simulink library "TriphaseHardwaremodule"  (R2019b)
settings: Solver=ode45  StartTime=0.0  StopTime=10.0  RelTol=1e-3
values from neighbouring files (symbols this model uses):
  ControlSampleTime = 1/8000    (= 0.000125)    [initTPHardware.m]
  HWSampleTime = ControlSampleTime / Oversample    [Sim_TP3_VSM_init.m]    (also in initTPHardware.m = 3.125e-05)
  L1 = 0    [initVirtualCircuit.m]
undefined symbols (not defined in the file or in its folder): C1, C2, C_cap, C_CM, C_damp, C_DC, DT, gcbh, Iac_bit, Iac_max, L2, L_CM, LCL, PWM_f, R_C1, R_C2, R_cap, R_damp, R_L1, R_L2, sps_rtmsupport, Vac_bit, Vac_max, Vdc_bit, Vdc_max
libraries: $bdroot x58, powerlib x46, triphase_hpc x7, powerlib_meascontrol x5, simulink x2
(part 2 of 3)

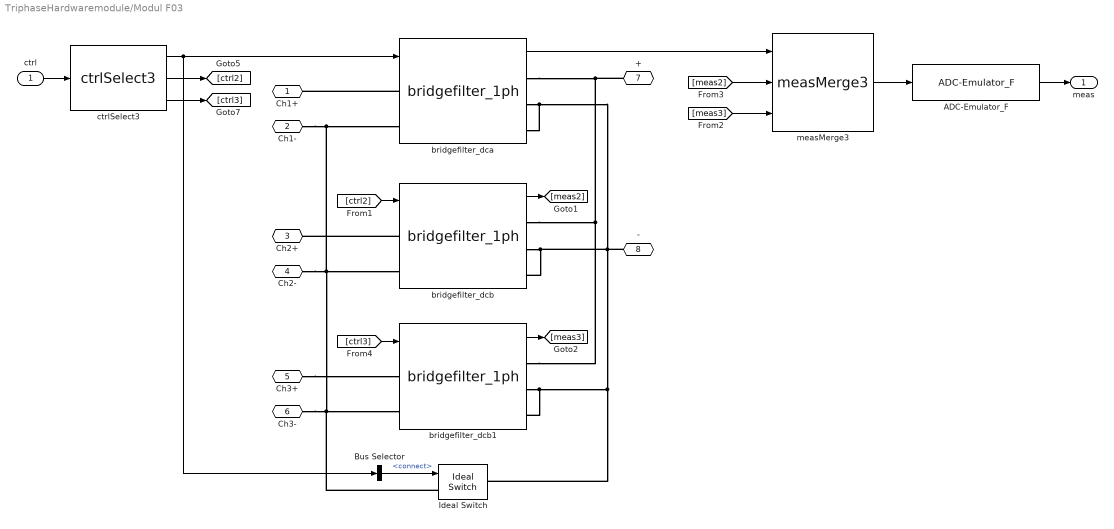
== system TriphaseHardwaremodule/Modul F03 ==
  ctrl : Inport
  ADC-Emulator_F : $bdroot/ADC-Emulator_F  ADC_Emulation=off  ControlSampleTime=ControlSampleTime  HWSampleTime=HWSampleTime  Vac_max=Vac_max  Vac_bit=Vac_bit  Iac_max=Iac_max  Iac_bit=Iac_bit  Vdc_max=Vdc_max  Vdc_bit=Vdc_bit
  Bus Selector : BusSelector  OutputSignals=connect
  Ideal Switch : powerlib/Power Electronics/Ideal Switch  Ron=0.001  Lon=0  IC=0  Rs=1e6  Cs=inf  Measurements=off
      settings: SourceProductName=Simscape Electrical
  bridgefilter_dca : $bdroot/bridgefilter_1ph  LCFilterChoice=LC  L1=L1  R_L1=R_L1  C1=C1  R_C1=R_C1  L2=L2  R_L2=R_L2  C2=C2  R_C2=R_C2  PWM_f=PWM_f  DT=DT
  bridgefilter_dcb : $bdroot/bridgefilter_1ph  LCFilterChoice=LC  L1=L1  R_L1=R_L1  C1=C1  R_C1=R_C1  L2=L2  R_L2=R_L2  C2=C2  R_C2=R_C2  PWM_f=PWM_f  DT=DT
  bridgefilter_dcb1 : $bdroot/bridgefilter_1ph  LCFilterChoice=LC  L1=L1  R_L1=R_L1  C1=C1  R_C1=R_C1  L2=L2  R_L2=R_L2  C2=C2  R_C2=R_C2  PWM_f=PWM_f  DT=DT
  ctrlSelect3 : $bdroot/ctrlSelect3
  measMerge3 : $bdroot/measMerge3
  Ch1+ : PMIOPort  Tag=PMCPort  Side=Left
  Ch1- : PMIOPort  Tag=PMCPort  Port=2  Side=Left
  Ch2+ : PMIOPort  Tag=PMCPort  Port=3  Side=Left
  Ch2- : PMIOPort  Tag=PMCPort  Port=4  Side=Left
  Ch3+ : PMIOPort  Tag=PMCPort  Port=5  Side=Left
  Ch3- : PMIOPort  Tag=PMCPort  Port=6  Side=Left
  + : PMIOPort  Tag=PMCPort  Port=7  Side=Right
  - : PMIOPort  Tag=PMCPort  Port=8  Side=Right
  meas : Outport  VectorParamsAs1DForOutWhenUnconnected=off
  wires:
  ADC-Emulator_F/1 -> meas/1
  measMerge3/1 -> ADC-Emulator_F/1
  Bus Selector/1 -> Ideal Switch/1  "<connect>"
  ctrlSelect3/1 -> bridgefilter_dca/1, Bus Selector/1
  bridgefilter_dcb/1 -> [meas2]
  bridgefilter_dca/1 -> measMerge3/1
  [meas2] -> measMerge3/2
  ctrl/1 -> ctrlSelect3/1
  ctrlSelect3/2 -> [ctrl2]
  [ctrl2] -> bridgefilter_dcb/1
  bridgefilter_dcb1/1 -> [meas3]
  [meas3] -> measMerge3/3
  ctrlSelect3/3 -> [ctrl3]
  [ctrl3] -> bridgefilter_dcb1/1
  connections:
  bridgefilter_dcb1/RConn2 -- bridgefilter_dcb1/RConn3 -- Ideal Switch/RConn1 -- -/RConn1 -- bridgefilter_dca/RConn3 -- bridgefilter_dca/RConn2 -- bridgefilter_dcb/RConn3 -- bridgefilter_dcb/RConn2
  +/RConn1 -- bridgefilter_dcb1/RConn1 -- bridgefilter_dcb/RConn1 -- bridgefilter_dca/RConn1
  bridgefilter_dcb/LConn1 -- Ch2+/RConn1
  bridgefilter_dca/LConn1 -- Ch1+/RConn1
  Ch3+/RConn1 -- bridgefilter_dcb1/LConn1
  Ch2-/RConn1 -- Ideal Switch/LConn1 -- Ch3-/RConn1 -- bridgefilter_dcb1/LConn2 -- bridgefilter_dcb/LConn2 -- Ch1-/RConn1 -- bridgefilter_dca/LConn2

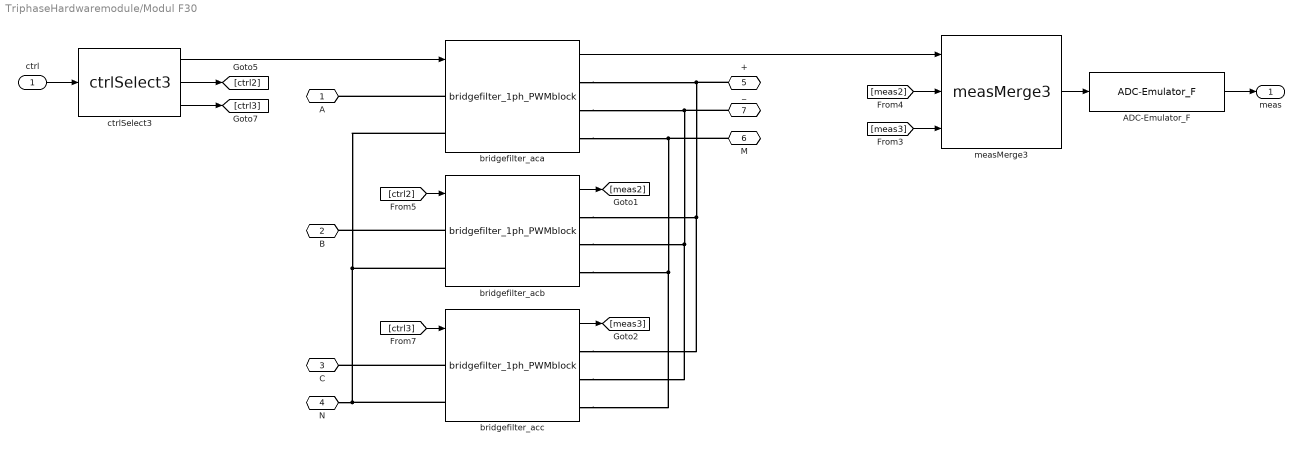
== system TriphaseHardwaremodule/Modul F30 ==
  ctrl : Inport
  ADC-Emulator_F : $bdroot/ADC-Emulator_F  ADC_Emulation=off  ControlSampleTime=ControlSampleTime  HWSampleTime=HWSampleTime  Vac_max=Vac_max  Vac_bit=Vac_bit  Iac_max=Iac_max  Iac_bit=Iac_bit  Vdc_max=Vdc_max  Vdc_bit=Vdc_bit
  bridgefilter_aca : $bdroot/bridgefilter_1ph_PWMblock  LCFilterChoice=LCLC  L1=L1  R_L1=R_L1  C1=C1  R_C1=R_C1  L2=L2  R_L2=R_L2  C2=C2  R_C2=R_C2  PWM_f=PWM_f  DT=DT  I_MAX=250  I_BACK=180
  bridgefilter_acb : $bdroot/bridgefilter_1ph_PWMblock  LCFilterChoice=LCLC  L1=L1  R_L1=R_L1  C1=C1  R_C1=R_C1  L2=L2  R_L2=R_L2  C2=C2  R_C2=R_C2  PWM_f=PWM_f  DT=DT  I_MAX=250  I_BACK=180
  bridgefilter_acc : $bdroot/bridgefilter_1ph_PWMblock  LCFilterChoice=LCLC  L1=L1  R_L1=R_L1  C1=C1  R_C1=R_C1  L2=L2  R_L2=R_L2  C2=C2  R_C2=R_C2  PWM_f=PWM_f  DT=DT  I_MAX=250  I_BACK=180
  ctrlSelect3 : $bdroot/ctrlSelect3  SystemSampleTime=-1
  measMerge3 : $bdroot/measMerge3  SystemSampleTime=-1
  A : PMIOPort  Tag=PMCPort  Side=Left
  B : PMIOPort  Tag=PMCPort  Port=2  Side=Left
  C : PMIOPort  Tag=PMCPort  Port=3  Side=Left
  N : PMIOPort  Tag=PMCPort  Port=4  Side=Left
  + : PMIOPort  Tag=PMCPort  Port=5  Side=Right
  M : PMIOPort  Tag=PMCPort  Port=6  Side=Right
  _ : PMIOPort  Tag=PMCPort  Port=7  Side=Right
  meas : Outport  VectorParamsAs1DForOutWhenUnconnected=off
  wires:
  measMerge3/1 -> ADC-Emulator_F/1
  ADC-Emulator_F/1 -> meas/1
  ctrlSelect3/1 -> bridgefilter_aca/1
  [ctrl3] -> bridgefilter_acc/1
  [ctrl2] -> bridgefilter_acb/1
  ctrlSelect3/2 -> [ctrl2]
  ctrlSelect3/3 -> [ctrl3]
  ctrl/1 -> ctrlSelect3/1
  [meas2] -> measMerge3/2
  bridgefilter_acc/1 -> [meas3]
  bridgefilter_acb/1 -> [meas2]
  [meas3] -> measMerge3/3
  bridgefilter_aca/1 -> measMerge3/1
  connections:
  bridgefilter_acc/LConn2 -- N/RConn1 -- bridgefilter_acb/LConn2 -- bridgefilter_aca/LConn2
  _/RConn1 -- bridgefilter_aca/RConn2 -- bridgefilter_acc/RConn2 -- bridgefilter_acb/RConn2
  bridgefilter_aca/RConn3 -- M/RConn1 -- bridgefilter_acc/RConn3 -- bridgefilter_acb/RConn3
  bridgefilter_aca/RConn1 -- +/RConn1 -- bridgefilter_acc/RConn1 -- bridgefilter_acb/RConn1
  bridgefilter_acc/LConn1 -- C/RConn1
  bridgefilter_acb/LConn1 -- B/RConn1
  bridgefilter_aca/LConn1 -- A/RConn1

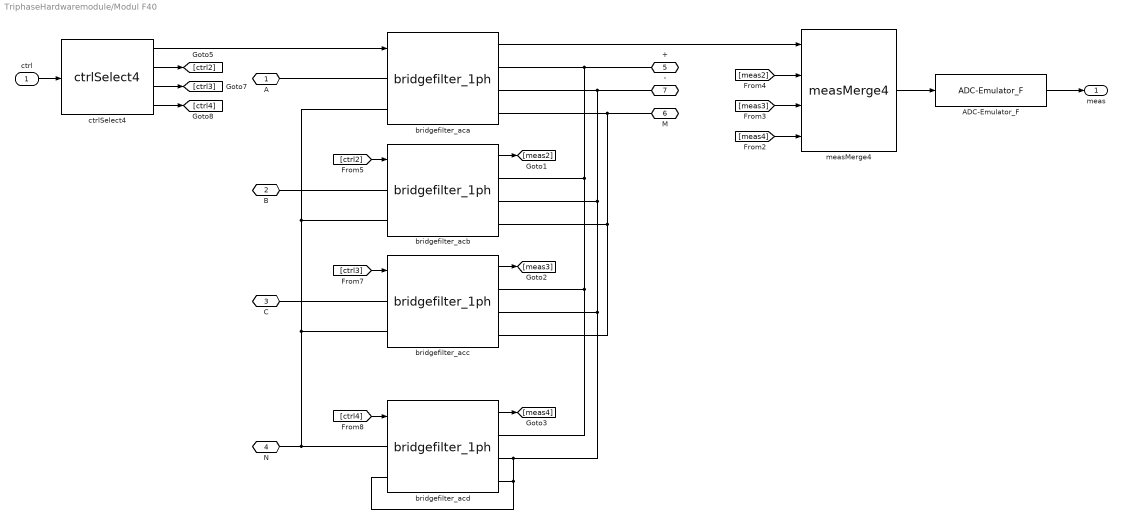
== system TriphaseHardwaremodule/Modul F40 ==
  ctrl : Inport
  ADC-Emulator_F : $bdroot/ADC-Emulator_F  ADC_Emulation=off  ControlSampleTime=ControlSampleTime  HWSampleTime=HWSampleTime  Vac_max=Vac_max  Vac_bit=Vac_bit  Iac_max=Iac_max  Iac_bit=Iac_bit  Vdc_max=Vdc_max  Vdc_bit=Vdc_bit
  bridgefilter_aca : $bdroot/bridgefilter_1ph  LCFilterChoice=LC  L1=L1  R_L1=R_L1  C1=C1  R_C1=R_C1  L2=L2  R_L2=R_L2  C2=C2  R_C2=R_C2  PWM_f=PWM_f  DT=DT
  bridgefilter_acb : $bdroot/bridgefilter_1ph  LCFilterChoice=LC  L1=L1  R_L1=R_L1  C1=C1  R_C1=R_C1  L2=L2  R_L2=R_L2  C2=C2  R_C2=R_C2  PWM_f=PWM_f  DT=DT
  bridgefilter_acc : $bdroot/bridgefilter_1ph  LCFilterChoice=LC  L1=L1  R_L1=R_L1  C1=C1  R_C1=R_C1  L2=L2  R_L2=R_L2  C2=C2  R_C2=R_C2  PWM_f=PWM_f  DT=DT
  bridgefilter_acd : $bdroot/bridgefilter_1ph  LCFilterChoice=LC  L1=L1  R_L1=R_L1  C1=C1  R_C1=R_C1  L2=L2  R_L2=R_L2  C2=C2  R_C2=R_C2  PWM_f=PWM_f  DT=DT
  ctrlSelect4 : $bdroot/ctrlSelect4
  measMerge4 : $bdroot/measMerge4
  A : PMIOPort  Tag=PMCPort  Side=Left
  B : PMIOPort  Tag=PMCPort  Port=2  Side=Left
  C : PMIOPort  Tag=PMCPort  Port=3  Side=Left
  N : PMIOPort  Tag=PMCPort  Port=4  Side=Left
  + : PMIOPort  Tag=PMCPort  Port=5  Side=Right
  M : PMIOPort  Tag=PMCPort  Port=6  Side=Right
  - : PMIOPort  Tag=PMCPort  Port=7  Side=Right
  meas : Outport  VectorParamsAs1DForOutWhenUnconnected=off
  wires:
  ctrlSelect4/1 -> bridgefilter_aca/1
  [ctrl4] -> bridgefilter_acd/1
  [ctrl3] -> bridgefilter_acc/1
  [ctrl2] -> bridgefilter_acb/1
  ctrlSelect4/2 -> [ctrl2]
  ctrlSelect4/3 -> [ctrl3]
  ctrlSelect4/4 -> [ctrl4]
  ctrl/1 -> ctrlSelect4/1
  measMerge4/1 -> ADC-Emulator_F/1
  [meas2] -> measMerge4/2
  bridgefilter_acd/1 -> [meas4]
  bridgefilter_acc/1 -> [meas3]
  bridgefilter_acb/1 -> [meas2]
  [meas4] -> measMerge4/4
  [meas3] -> measMerge4/3
  bridgefilter_aca/1 -> measMerge4/1
  ADC-Emulator_F/1 -> meas/1
  connections:
  bridgefilter_acc/LConn2 -- N/RConn1 -- bridgefilter_acd/LConn1 -- bridgefilter_acb/LConn2 -- bridgefilter_aca/LConn2
  bridgefilter_acc/LConn1 -- C/RConn1
  bridgefilter_acb/LConn1 -- B/RConn1
  bridgefilter_aca/LConn1 -- A/RConn1
  bridgefilter_aca/RConn1 -- bridgefilter_acd/RConn1 -- bridgefilter_acc/RConn1 -- bridgefilter_acb/RConn1 -- +/RConn1
  -/RConn1 -- bridgefilter_aca/RConn2 -- bridgefilter_acb/RConn2 -- bridgefilter_acd/LConn2 -- bridgefilter_acd/RConn3 -- bridgefilter_acd/RConn2 -- bridgefilter_acc/RConn2
  M/RConn1 -- bridgefilter_acc/RConn3 -- bridgefilter_acb/RConn3 -- bridgefilter_aca/RConn3

== system TriphaseHardwaremodule/Modul M30 ==
  ctrl : Inport
  ADC-Emulator_M : $bdroot/ADC-Emulator_M  ADC_Emulation=off  ControlSampleTime=ControlSampleTime  HWSampleTime=HWSampleTime  Vac_max=Vac_max  Vac_bit=Vac_bit  Iac_max=Iac_max  Iac_bit=Iac_bit  Vdc_max=Vdc_max  Vdc_bit=Vdc_bit
  B6 Brücke : Subsystem  InitFcn=|  Variant=on
      | if ~exist('SimulationMode','var')
      | SimulationMode = 1;
      | end
      settings: AttributesFormatString=%<ActiveVariant>
  Bus Creator : BusCreator  Inputs=2
  Bus Selector : BusSelector  OutputSignals=pwm
  Decoupling Resistance : powerlib/Elements/Three-Phase Parallel RLC Branch  LConnTagsString=A|B|C  RConnTagsString=A|B|C  BranchType=R  Resistance=0.0001  Inductance=1e-3  Capacitance=1e-6  Measurements=None
      settings: SourceProductName=Simscape Electrical  SourceProductBaseCode=PS
  Three-Phase I-Measurement (right to left = positive) : powerlib/Measurements/Three-Phase V-I Measurement  VoltageMeasurement=no  SetLabelV=off  LabelV=Vabc  Vpu=off  VpuLL=off  CurrentMeasurement=yes  SetLabelI=off  LabelI=I_out  Ipu=off  Pbase=100e6  Vbase=500e3  OutputType=Complex  PhasorSimulation=off  PSBequivalent=0
      settings: SourceProductName=Simscape Electrical
  Voltage Measurement : powerlib/Measurements/Voltage Measurement  PhasorSimulation=off  OutputType=Complex  PSBequivalent=0
      settings: SourceProductName=Simscape Electrical
  + : PMIOPort  Side=Right
  - : PMIOPort  Port=2  Side=Right
  A : PMIOPort  Port=3  Side=Left
  B : PMIOPort  Port=4  Side=Left
  C : PMIOPort  Port=5  Side=Left
  meas : Outport  VectorParamsAs1DForOutWhenUnconnected=off
  wires:
  Three-Phase I-Measurement (right to left = positive)/1 -> Bus Creator/1  "meas_i_inverter"
  Voltage Measurement/1 -> Bus Creator/2  "meas_u_dc"
  ctrl/1 -> Bus Selector/1
  Bus Selector/1 -> B6 Brücke/1(DutyCycle)  "<pwm>"
  Bus Creator/1 -> ADC-Emulator_M/1
  ADC-Emulator_M/1 -> meas/1
  connections:
  -/RConn1 -- Voltage Measurement/LConn2 -- B6 Brücke/RConn2
  B6 Brücke/RConn1 -- Voltage Measurement/LConn1 -- +/RConn1
  Three-Phase I-Measurement (right to left = positive)/LConn1 -- B6 Brücke/LConn1
  Three-Phase I-Measurement (right to left = positive)/LConn2 -- B6 Brücke/LConn2
  Three-Phase I-Measurement (right to left = positive)/LConn3 -- B6 Brücke/LConn3
  Decoupling Resistance/RConn3 -- Three-Phase I-Measurement (right to left = positive)/RConn3
  Decoupling Resistance/RConn2 -- Three-Phase I-Measurement (right to left = positive)/RConn2
  Decoupling Resistance/RConn1 -- Three-Phase I-Measurement (right to left = positive)/RConn1
  A/RConn1 -- Decoupling Resistance/LConn1
  B/RConn1 -- Decoupling Resistance/LConn2
  C/RConn1 -- Decoupling Resistance/LConn3

== system TriphaseHardwaremodule/PMXXF03C ==
  Setpoints : Inport
  Bus Creator : BusCreator  Inputs=1
  Bus Selector : BusSelector  OutputSignals=preload,Inv1
  DC-Bus : $bdroot/DC-Bus  C_cap=C_cap  R_cap=R_cap
  Modul F03 : $bdroot/Modul F03  Leistungsklasse=Custom  LCFilterChoice=LC  L1=L1  R_L1=R_L1  C1=C1  R_C1=R_C1  L2=L2  R_L2=R_L2  C2=C2  R_C2=R_C2  PWM_f=PWM_f  DT=DT  ADC_Emulation=off  ControlSampleTime=ControlSampleTime  HWSampleTime=HWSampleTime  Vac_max=Vac_max  Vac_bit=Vac_bit  Iac_max=Iac_max  Iac_bit=Iac_bit  Vdc_max=Vdc_max  Vdc_bit=Vdc_bit
  A1+ : PMIOPort  Tag=PMCPort  Side=Left
  A1- : PMIOPort  Tag=PMCPort  Port=2  Side=Left
  B1+ : PMIOPort  Tag=PMCPort  Port=3  Side=Left
  B1- : PMIOPort  Tag=PMCPort  Port=4  Side=Left
  C1+ : PMIOPort  Tag=PMCPort  Port=5  Side=Left
  C1- : PMIOPort  Tag=PMCPort  Port=6  Side=Left
  A_rect : PMIOPort  Tag=PMCPort  Port=7  Side=Right
  B_rect : PMIOPort  Tag=PMCPort  Port=8  Side=Right
  C_rect : PMIOPort  Tag=PMCPort  Port=9  Side=Right
  ZWK+ : PMIOPort  Tag=PMCPort  Port=10  Side=Right
  ZWK- : PMIOPort  Tag=PMCPort  Port=11  Side=Right
  Measurements : Outport  VectorParamsAs1DForOutWhenUnconnected=off
  wires:
  Setpoints/1 -> Bus Selector/1
  Bus Selector/1 -> DC-Bus/1  "<preload>"
  Bus Creator/1 -> Measurements/1
  Modul F03/1 -> Bus Creator/1  "Inv1"
  Bus Selector/2 -> Modul F03/1  "<Inv1>"
  connections:
  Modul F03/RConn1 -- DC-Bus/LConn4
  Modul F03/LConn1 -- A1+/RConn1
  DC-Bus/RConn1 -- A_rect/RConn1
  DC-Bus/RConn2 -- B_rect/RConn1
  DC-Bus/RConn3 -- C_rect/RConn1
  ZWK+/RConn1 -- DC-Bus/RConn4
  DC-Bus/RConn5 -- ZWK-/RConn1
  Modul F03/RConn2 -- DC-Bus/LConn6
  A1-/RConn1 -- Modul F03/LConn2
  B1+/RConn1 -- Modul F03/LConn3
  B1-/RConn1 -- Modul F03/LConn4
  C1+/RConn1 -- Modul F03/LConn5
  C1-/RConn1 -- Modul F03/LConn6

== system TriphaseHardwaremodule/PMXXF30C ==
  Setpoints : Inport
  Bus Creator : BusCreator  Inputs=1
  Bus Selector : BusSelector  OutputSignals=preload,Inv1
  DC-Bus : $bdroot/DC-Bus  C_cap=C_cap  R_cap=R_cap
  Modul F30 : $bdroot/Modul F30  Leistungsklasse=Custom  LCFilterChoice=LC  L1=L1  R_L1=R_L1  C1=C1  R_C1=R_C1  L2=L2  R_L2=R_L2  C2=C2  R_C2=R_C2  PWM_f=PWM_f  DT=DT  ADC_Emulation=off  ControlSampleTime=ControlSampleTime  HWSampleTime=HWSampleTime  Vac_max=Vac_max  Vac_bit=Vac_bit  Iac_max=Iac_max  Iac_bit=Iac_bit  Vdc_max=Vdc_max  Vdc_bit=Vdc_bit
  A1 : PMIOPort  Tag=PMCPort  Side=Left
  B1 : PMIOPort  Tag=PMCPort  Port=2  Side=Left
  C1 : PMIOPort  Tag=PMCPort  Port=3  Side=Left
  N1 : PMIOPort  Tag=PMCPort  Port=4  Side=Left
  A_rect : PMIOPort  Tag=PMCPort  Port=5  Side=Right
  B_rect : PMIOPort  Tag=PMCPort  Port=6  Side=Right
  C_rect : PMIOPort  Tag=PMCPort  Port=7  Side=Right
  ZWK+ : PMIOPort  Tag=PMCPort  Port=8  Side=Right
  ZWK- : PMIOPort  Tag=PMCPort  Port=9  Side=Right
  Measurements : Outport  VectorParamsAs1DForOutWhenUnconnected=off
  wires:
  Bus Selector/2 -> Modul F30/1  "<Inv1>"
  Setpoints/1 -> Bus Selector/1
  Bus Selector/1 -> DC-Bus/1  "<preload>"
  Bus Creator/1 -> Measurements/1
  Modul F30/1 -> Bus Creator/1  "Inv1"
  connections:
  Modul F30/LConn3 -- C1/RConn1
  Modul F30/LConn2 -- B1/RConn1
  Modul F30/LConn1 -- A1/RConn1
  DC-Bus/LConn1 -- Modul F30/RConn1
  DC-Bus/LConn2 -- Modul F30/RConn2
  DC-Bus/LConn3 -- Modul F30/RConn3
  DC-Bus/RConn3 -- C_rect/RConn1
  DC-Bus/RConn2 -- B_rect/RConn1
  DC-Bus/RConn1 -- A_rect/RConn1
  DC-Bus/RConn4 -- ZWK+/RConn1
  DC-Bus/RConn5 -- ZWK-/RConn1
  N1/RConn1 -- Modul F30/LConn4

== system TriphaseHardwaremodule/PMXXF30Cver270612 ==
  Setpoints : Inport
  Bus Creator : BusCreator  Inputs=2
  Bus Selector : BusSelector  OutputSignals=preload,Inv1
  DC-Bus : $bdroot/DC-Bus  C_cap=C_cap  R_cap=R_cap
  Modul F30 : $bdroot/Modul F30  Leistungsklasse=Custom  LCFilterChoice=LC  L1=L1  R_L1=R_L1  C1=C1  R_C1=R_C1  L2=L2  R_L2=R_L2  C2=C2  R_C2=R_C2  PWM_f=PWM_f  DT=DT  ADC_Emulation=off  ControlSampleTime=ControlSampleTime  HWSampleTime=HWSampleTime  Vac_max=Vac_max  Vac_bit=Vac_bit  Iac_max=Iac_max  Iac_bit=Iac_bit  Vdc_max=Vdc_max  Vdc_bit=Vdc_bit
  emptyMeasure : $bdroot/emptyMeasure
  A1 : PMIOPort  Tag=PMCPort  Side=Left
  B1 : PMIOPort  Tag=PMCPort  Port=2  Side=Left
  C1 : PMIOPort  Tag=PMCPort  Port=3  Side=Left
  N1 : PMIOPort  Tag=PMCPort  Port=4  Side=Left
  ZWK+ : PMIOPort  Tag=PMCPort  Port=5  Side=Right
  ZWK- : PMIOPort  Tag=PMCPort  Port=6  Side=Right
  Measurements : Outport  VectorParamsAs1DForOutWhenUnconnected=off
  wires:
  Bus Selector/1 -> DC-Bus/1  "<preload>"
  Setpoints/1 -> Bus Selector/1
  Bus Creator/1 -> Measurements/1
  Modul F30/1 -> Bus Creator/1  "Inv1"
  emptyMeasure/1 -> Bus Creator/2  "Inv2"
  Bus Selector/2 -> Modul F30/1  "<Inv1>"
  connections:
  DC-Bus/RConn1 -- Modul F30/LConn1 -- A1/RConn1
  DC-Bus/RConn2 -- B1/RConn1 -- Modul F30/LConn2
  DC-Bus/RConn3 -- Modul F30/LConn3 -- C1/RConn1
  ZWK-/RConn1 -- DC-Bus/RConn5
  ZWK+/RConn1 -- DC-Bus/RConn4
  Modul F30/RConn1 -- DC-Bus/LConn1
  Modul F30/RConn2 -- DC-Bus/LConn2
  Modul F30/RConn3 -- DC-Bus/LConn3
  N1/RConn1 -- Modul F30/LConn4

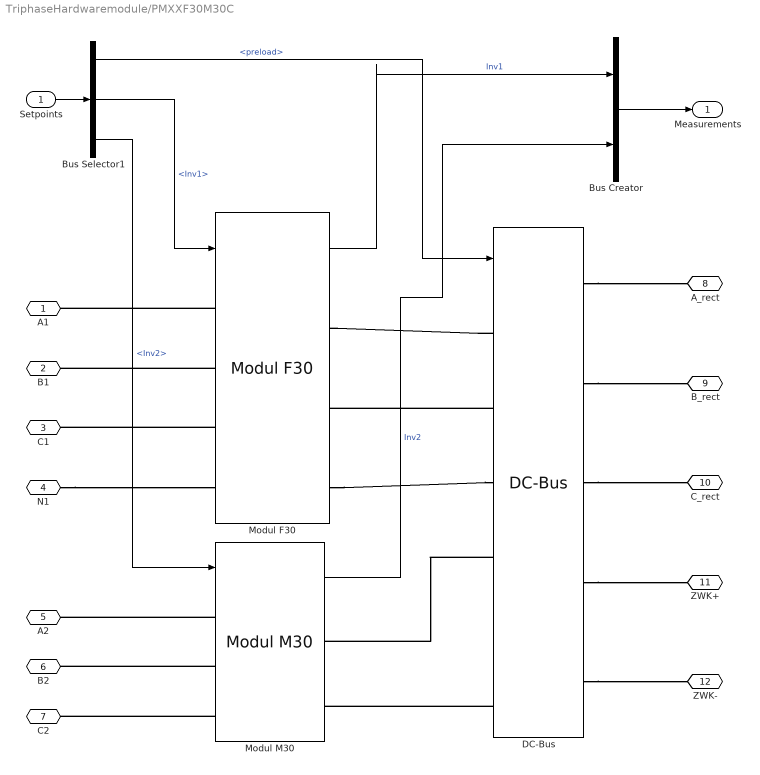
== system TriphaseHardwaremodule/PMXXF30M30C ==
  Setpoints : Inport
  Bus Creator : BusCreator  Inputs=2
  Bus Selector1 : BusSelector  OutputSignals=preload,Inv1,Inv2
  DC-Bus : $bdroot/DC-Bus  C_cap=C_cap  R_cap=R_cap
  Modul F30 : $bdroot/Modul F30  Leistungsklasse=Custom  LCFilterChoice=LC  L1=L1  R_L1=R_L1  C1=C1  R_C1=R_C1  L2=L2  R_L2=R_L2  C2=C2  R_C2=R_C2  PWM_f=PWM_f  DT=DT  ADC_Emulation=off  ControlSampleTime=ControlSampleTime  HWSampleTime=HWSampleTime  Vac_max=Vac_max  Vac_bit=Vac_bit  Iac_max=Iac_max  Iac_bit=Iac_bit  Vdc_max=Vdc_max  Vdc_bit=Vdc_bit
  Modul M30 : $bdroot/Modul M30  PWM_f=PWM_f  DT=DT
  A1 : PMIOPort  Tag=PMCPort  Side=Left
  B1 : PMIOPort  Tag=PMCPort  Port=2  Side=Left
  C1 : PMIOPort  Tag=PMCPort  Port=3  Side=Left
  N1 : PMIOPort  Tag=PMCPort  Port=4  Side=Left
  A2 : PMIOPort  Tag=PMCPort  Port=5  Side=Left
  B2 : PMIOPort  Tag=PMCPort  Port=6  Side=Left
  C2 : PMIOPort  Tag=PMCPort  Port=7  Side=Left
  A_rect : PMIOPort  Tag=PMCPort  Port=8  Side=Right
  B_rect : PMIOPort  Tag=PMCPort  Port=9  Side=Right
  C_rect : PMIOPort  Tag=PMCPort  Port=10  Side=Right
  ZWK+ : PMIOPort  Tag=PMCPort  Port=11  Side=Right
  ZWK- : PMIOPort  Tag=PMCPort  Port=12  Side=Right
  Measurements : Outport  VectorParamsAs1DForOutWhenUnconnected=off
  wires:
  Bus Selector1/3 -> Modul M30/1  "<Inv2>"
  Bus Selector1/2 -> Modul F30/1  "<Inv1>"
  Setpoints/1 -> Bus Selector1/1
  Modul F30/1 -> Bus Creator/1  "Inv1"
  Bus Selector1/1 -> DC-Bus/1  "<preload>"
  Bus Creator/1 -> Measurements/1
  Modul M30/1 -> Bus Creator/2  "Inv2"
  connections:
  Modul F30/LConn3 -- C1/RConn1
  Modul F30/LConn2 -- B1/RConn1
  Modul F30/LConn1 -- A1/RConn1
  Modul M30/LConn2 -- B2/RConn1
  Modul M30/LConn1 -- A2/RConn1
  Modul M30/LConn3 -- C2/RConn1
  DC-Bus/RConn3 -- C_rect/RConn1
  DC-Bus/RConn2 -- B_rect/RConn1
  DC-Bus/RConn1 -- A_rect/RConn1
  DC-Bus/RConn4 -- ZWK+/RConn1
  DC-Bus/RConn5 -- ZWK-/RConn1
  DC-Bus/LConn2 -- Modul F30/RConn2
  DC-Bus/LConn1 -- Modul F30/RConn1
  DC-Bus/LConn4 -- Modul M30/RConn1
  DC-Bus/LConn6 -- Modul M30/RConn2
  Modul F30/RConn3 -- DC-Bus/LConn3
  N1/RConn1 -- Modul F30/LConn4

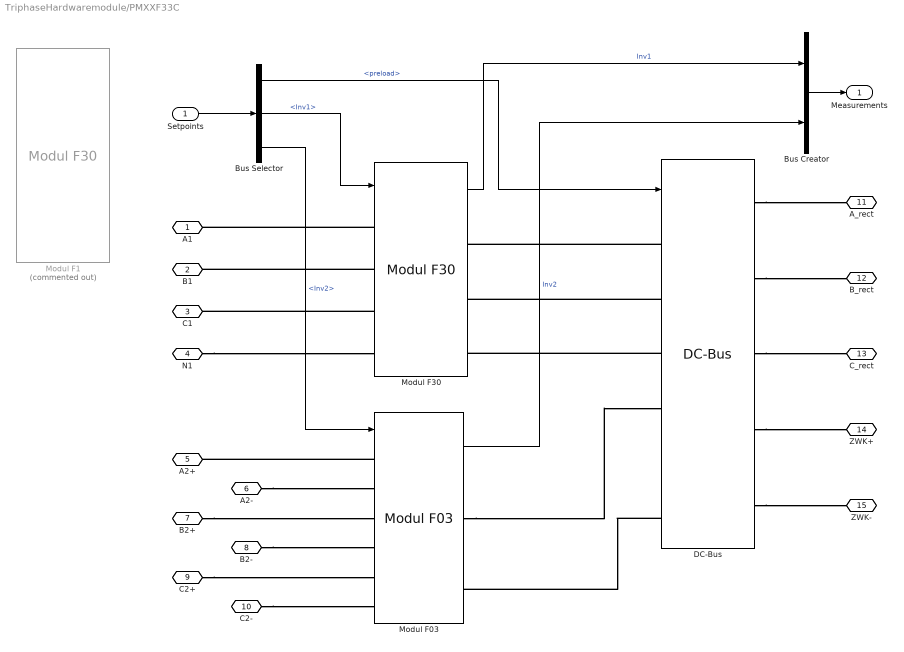
== system TriphaseHardwaremodule/PMXXF33C ==
  Setpoints : Inport
  Bus Creator : BusCreator  Inputs=2
  Bus Selector : BusSelector  OutputSignals=preload,Inv1,Inv2
  DC-Bus : $bdroot/DC-Bus  C_cap=C_cap  R_cap=R_cap
  Modul F03 : $bdroot/Modul F03  Leistungsklasse=Custom  LCFilterChoice=LC  L1=L1  R_L1=R_L1  C1=C1  R_C1=R_C1  L2=L2  R_L2=R_L2  C2=C2  R_C2=R_C2  PWM_f=PWM_f  DT=DT  ADC_Emulation=off  ControlSampleTime=ControlSampleTime  HWSampleTime=HWSampleTime  Vac_max=Vac_max  Vac_bit=Vac_bit  Iac_max=Iac_max  Iac_bit=Iac_bit  Vdc_max=Vdc_max  Vdc_bit=Vdc_bit
  Modul F1 : $bdroot/Modul F30  Commented=on  Leistungsklasse=Custom  LCFilterChoice=LCLC  L1=L1  R_L1=R_L1  C1=C1  R_C1=R_C1  L2=L2  R_L2=R_L2  C2=C2  R_C2=R_C2  PWM_f=PWM_f  DT=DT  ADC_Emulation=off  ControlSampleTime=ControlSampleTime  HWSampleTime=HWSampleTime  Vac_max=Vac_max  Vac_bit=Vac_bit  Iac_max=Iac_max  Iac_bit=Iac_bit  Vdc_max=Vdc_max  Vdc_bit=Vdc_bit
  Modul F30 : $bdroot/Modul F30  Leistungsklasse=Custom  LCFilterChoice=LCLC  L1=L1  R_L1=R_L1  C1=C1  R_C1=R_C1  L2=L2  R_L2=R_L2  C2=C2  R_C2=R_C2  PWM_f=PWM_f  DT=DT  ADC_Emulation=off  ControlSampleTime=ControlSampleTime  HWSampleTime=HWSampleTime  Vac_max=Vac_max  Vac_bit=Vac_bit  Iac_max=Iac_max  Iac_bit=Iac_bit  Vdc_max=Vdc_max  Vdc_bit=Vdc_bit
  A1 : PMIOPort  Tag=PMCPort  Side=Left
  B1 : PMIOPort  Tag=PMCPort  Port=2  Side=Left
  C1 : PMIOPort  Tag=PMCPort  Port=3  Side=Left
  N1 : PMIOPort  Tag=PMCPort  Port=4  Side=Left
  A2+ : PMIOPort  Tag=PMCPort  Port=5  Side=Left
  A2- : PMIOPort  Tag=PMCPort  Port=6  Side=Left
  B2+ : PMIOPort  Tag=PMCPort  Port=7  Side=Left
  B2- : PMIOPort  Tag=PMCPort  Port=8  Side=Left
  C2+ : PMIOPort  Tag=PMCPort  Port=9  Side=Left
  C2- : PMIOPort  Tag=PMCPort  Port=10  Side=Left
  A_rect : PMIOPort  Tag=PMCPort  Port=11  Side=Right
  B_rect : PMIOPort  Tag=PMCPort  Port=12  Side=Right
  C_rect : PMIOPort  Tag=PMCPort  Port=13  Side=Right
  ZWK+ : PMIOPort  Tag=PMCPort  Port=14  Side=Right
  ZWK- : PMIOPort  Tag=PMCPort  Port=15  Side=Right
  Measurements : Outport  VectorParamsAs1DForOutWhenUnconnected=off
  wires:
  Setpoints/1 -> Bus Selector/1
  Bus Selector/2 -> Modul F30/1  "<Inv1>"
  Bus Selector/3 -> Modul F03/1  "<Inv2>"
  Bus Creator/1 -> Measurements/1
  Modul F30/1 -> Bus Creator/1  "Inv1"
  Modul F03/1 -> Bus Creator/2  "Inv2"
  Bus Selector/1 -> DC-Bus/1  "<preload>"
  connections:
  Modul F30/LConn1 -- A1/RConn1
  Modul F30/LConn2 -- B1/RConn1
  Modul F30/LConn3 -- C1/RConn1
  DC-Bus/RConn3 -- C_rect/RConn1
  Modul F03/LConn1 -- A2+/RConn1
  DC-Bus/RConn1 -- A_rect/RConn1
  DC-Bus/RConn2 -- B_rect/RConn1
  DC-Bus/RConn4 -- ZWK+/RConn1
  DC-Bus/RConn5 -- ZWK-/RConn1
  DC-Bus/LConn1 -- Modul F30/RConn1
  DC-Bus/LConn2 -- Modul F30/RConn2
  DC-Bus/LConn3 -- Modul F30/RConn3
  Modul F03/RConn1 -- DC-Bus/LConn4
  DC-Bus/LConn6 -- Modul F03/RConn2
  B2+/RConn1 -- Modul F03/LConn3
  C2+/RConn1 -- Modul F03/LConn5
  C2-/RConn1 -- Modul F03/LConn6
  A2-/RConn1 -- Modul F03/LConn2
  B2-/RConn1 -- Modul F03/LConn4
  N1/RConn1 -- Modul F30/LConn4

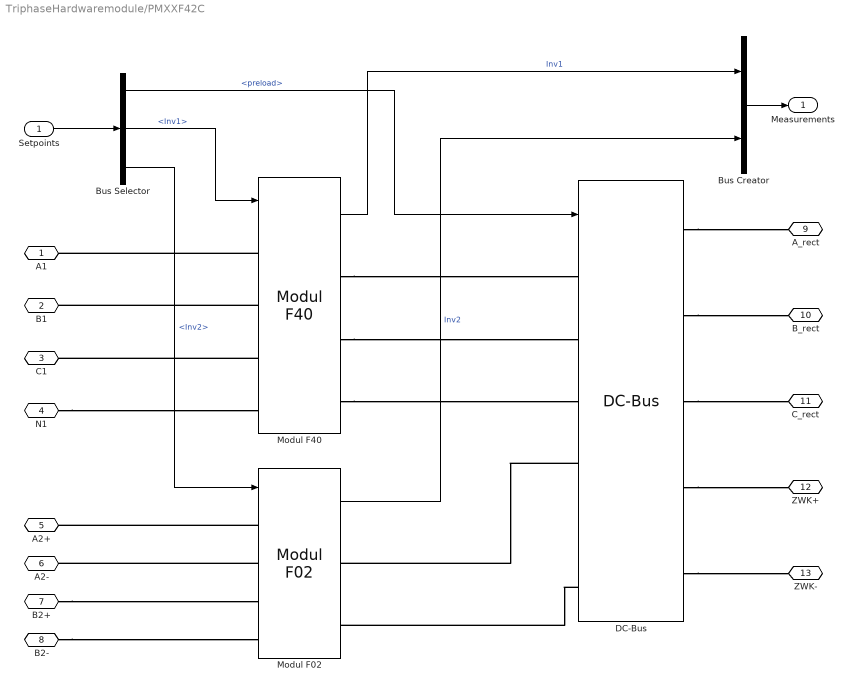
== system TriphaseHardwaremodule/PMXXF42C ==
  Setpoints : Inport
  Bus Creator : BusCreator  Inputs=2
  Bus Selector : BusSelector  OutputSignals=preload,Inv1,Inv2
  DC-Bus : $bdroot/DC-Bus  C_cap=C_cap  R_cap=R_cap
  Modul F02 : $bdroot/Modul F02  Leistungsklasse=Custom  LCFilterChoice=LC  L1=L1  R_L1=R_L1  C1=C1  R_C1=R_C1  L2=L2  R_L2=R_L2  C2=C2  R_C2=R_C2  PWM_f=PWM_f  DT=DT  ADC_Emulation=off  ControlSampleTime=ControlSampleTime  HWSampleTime=HWSampleTime  Vac_max=Vac_max  Vac_bit=Vac_bit  Iac_max=Iac_max  Iac_bit=Iac_bit  Vdc_max=Vdc_max  Vdc_bit=Vdc_bit
  Modul F40 : $bdroot/Modul F40  Leistungsklasse=Custom  LCFilterChoice=LC  L1=L1  R_L1=R_L1  C1=C1  R_C1=R_C1  L2=L2  R_L2=R_L2  C2=C2  R_C2=R_C2  PWM_f=PWM_f  DT=DT  ADC_Emulation=off  ControlSampleTime=ControlSampleTime  HWSampleTime=HWSampleTime  Vac_max=Vac_max  Vac_bit=Vac_bit  Iac_max=Iac_max  Iac_bit=Iac_bit  Vdc_max=Vdc_max  Vdc_bit=Vdc_bit
  A1 : PMIOPort  Tag=PMCPort  Side=Left
  B1 : PMIOPort  Tag=PMCPort  Port=2  Side=Left
  C1 : PMIOPort  Tag=PMCPort  Port=3  Side=Left
  N1 : PMIOPort  Tag=PMCPort  Port=4  Side=Left
  A2+ : PMIOPort  Tag=PMCPort  Port=5  Side=Left
  A2- : PMIOPort  Tag=PMCPort  Port=6  Side=Left
  B2+ : PMIOPort  Tag=PMCPort  Port=7  Side=Left
  B2- : PMIOPort  Tag=PMCPort  Port=8  Side=Left
  A_rect : PMIOPort  Tag=PMCPort  Port=9  Side=Right
  B_rect : PMIOPort  Tag=PMCPort  Port=10  Side=Right
  C_rect : PMIOPort  Tag=PMCPort  Port=11  Side=Right
  ZWK+ : PMIOPort  Tag=PMCPort  Port=12  Side=Right
  ZWK- : PMIOPort  Tag=PMCPort  Port=13  Side=Right
  Measurements : Outport  VectorParamsAs1DForOutWhenUnconnected=off
  wires:
  Bus Selector/1 -> DC-Bus/1  "<preload>"
  Modul F02/1 -> Bus Creator/2  "Inv2"
  Modul F40/1 -> Bus Creator/1  "Inv1"
  Bus Creator/1 -> Measurements/1
  Bus Selector/3 -> Modul F02/1  "<Inv2>"
  Bus Selector/2 -> Modul F40/1  "<Inv1>"
  Setpoints/1 -> Bus Selector/1
  connections:
  DC-Bus/LConn6 -- Modul F02/RConn2
  DC-Bus/LConn4 -- Modul F02/RConn1
  Modul F40/RConn3 -- DC-Bus/LConn3
  Modul F40/RConn2 -- DC-Bus/LConn2
  Modul F40/RConn1 -- DC-Bus/LConn1
  Modul F02/LConn2 -- A2-/RConn1
  DC-Bus/RConn5 -- ZWK-/RConn1
  DC-Bus/RConn4 -- ZWK+/RConn1
  DC-Bus/RConn2 -- B_rect/RConn1
  DC-Bus/RConn1 -- A_rect/RConn1
  Modul F02/LConn1 -- A2+/RConn1
  DC-Bus/RConn3 -- C_rect/RConn1
  Modul F40/LConn3 -- C1/RConn1
  Modul F40/LConn2 -- B1/RConn1
  Modul F40/LConn1 -- A1/RConn1
  N1/RConn1 -- Modul F40/LConn4
  B2+/RConn1 -- Modul F02/LConn3
  B2-/RConn1 -- Modul F02/LConn4

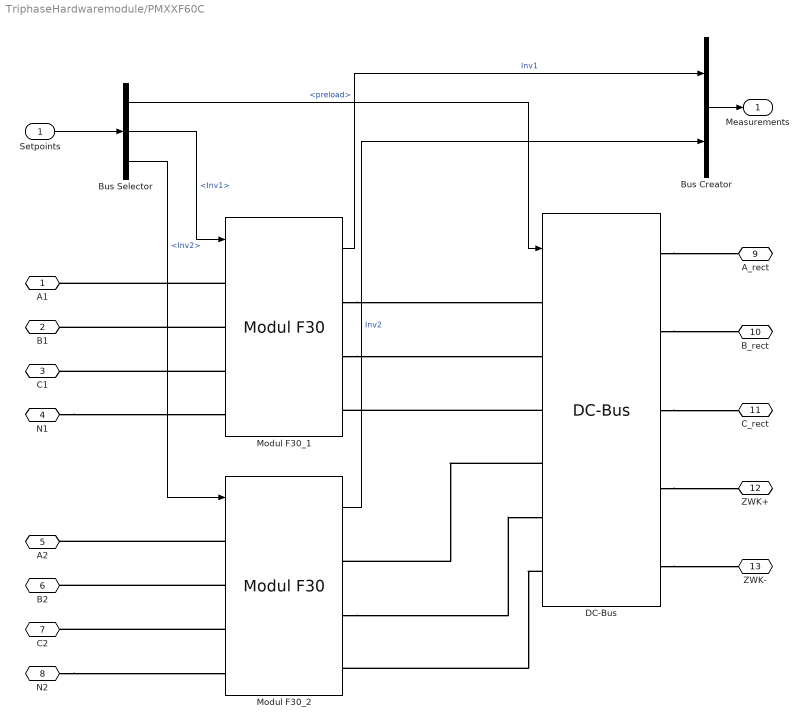
== system TriphaseHardwaremodule/PMXXF60C ==
  Setpoints : Inport
  Bus Creator : BusCreator  Inputs=2
  Bus Selector : BusSelector  OutputSignals=preload,Inv1,Inv2
  DC-Bus : $bdroot/DC-Bus  C_cap=C_cap  R_cap=R_cap
  Modul F30_1 : $bdroot/Modul F30  Leistungsklasse=Custom  LCFilterChoice=LC  L1=L1  R_L1=R_L1  C1=C1  R_C1=R_C1  L2=L2  R_L2=R_L2  C2=C2  R_C2=R_C2  PWM_f=PWM_f  DT=DT  ADC_Emulation=off  ControlSampleTime=ControlSampleTime  HWSampleTime=HWSampleTime  Vac_max=Vac_max  Vac_bit=Vac_bit  Iac_max=Iac_max  Iac_bit=Iac_bit  Vdc_max=Vdc_max  Vdc_bit=Vdc_bit
  Modul F30_2 : $bdroot/Modul F30  Leistungsklasse=Custom  LCFilterChoice=LC  L1=L1  R_L1=R_L1  C1=C1  R_C1=R_C1  L2=L2  R_L2=R_L2  C2=C2  R_C2=R_C2  PWM_f=PWM_f  DT=DT  ADC_Emulation=off  ControlSampleTime=ControlSampleTime  HWSampleTime=HWSampleTime  Vac_max=Vac_max  Vac_bit=Vac_bit  Iac_max=Iac_max  Iac_bit=Iac_bit  Vdc_max=Vdc_max  Vdc_bit=Vdc_bit
  A1 : PMIOPort  Tag=PMCPort  Side=Left
  "B1 " : PMIOPort  Tag=PMCPort  Port=2  Side=Left
  C1 : PMIOPort  Tag=PMCPort  Port=3  Side=Left
  N1 : PMIOPort  Tag=PMCPort  Port=4  Side=Left
  A2 : PMIOPort  Tag=PMCPort  Port=5  Side=Left
  B2 : PMIOPort  Tag=PMCPort  Port=6  Side=Left
  C2 : PMIOPort  Tag=PMCPort  Port=7  Side=Left
  N2 : PMIOPort  Tag=PMCPort  Port=8  Side=Left
  A_rect : PMIOPort  Tag=PMCPort  Port=9  Side=Right
  B_rect : PMIOPort  Tag=PMCPort  Port=10  Side=Right
  C_rect : PMIOPort  Tag=PMCPort  Port=11  Side=Right
  ZWK+ : PMIOPort  Tag=PMCPort  Port=12  Side=Right
  ZWK- : PMIOPort  Tag=PMCPort  Port=13  Side=Right
  Measurements : Outport  VectorParamsAs1DForOutWhenUnconnected=off
  wires:
  Setpoints/1 -> Bus Selector/1
  Bus Selector/3 -> Modul F30_2/1  "<Inv2>"
  Modul F30_1/1 -> Bus Creator/1  "Inv1"
  Modul F30_2/1 -> Bus Creator/2  "Inv2"
  Bus Selector/1 -> DC-Bus/1  "<preload>"
  Bus Creator/1 -> Measurements/1
  Bus Selector/2 -> Modul F30_1/1  "<Inv1>"
  connections:
  Modul F30_2/RConn2 -- DC-Bus/LConn5
  DC-Bus/LConn3 -- Modul F30_1/RConn3
  Modul F30_1/RConn2 -- DC-Bus/LConn2
  Modul F30_1/RConn1 -- DC-Bus/LConn1
  Modul F30_1/LConn1 -- A1/RConn1
  Modul F30_1/LConn2 -- "B1 "/RConn1
  Modul F30_1/LConn3 -- C1/RConn1
  Modul F30_2/LConn1 -- A2/RConn1
  Modul F30_2/LConn2 -- B2/RConn1
  Modul F30_2/LConn3 -- C2/RConn1
  DC-Bus/RConn3 -- C_rect/RConn1
  DC-Bus/RConn2 -- B_rect/RConn1
  DC-Bus/RConn1 -- A_rect/RConn1
  DC-Bus/RConn4 -- ZWK+/RConn1
  DC-Bus/RConn5 -- ZWK-/RConn1
  DC-Bus/LConn4 -- Modul F30_2/RConn1
  DC-Bus/LConn6 -- Modul F30_2/RConn3
  N1/RConn1 -- Modul F30_1/LConn4
  N2/RConn1 -- Modul F30_2/LConn4

== system TriphaseHardwaremodule/PWM delay AVG model4 ==
  In1 : Inport
  Average : Subsystem  TreatAsAtomicUnit=on
  Constant : Constant  Value=SIM_BRIDGE==SimBridgeMode.SWITCHED  SampleTime=HWSampleTime
  Logical Operator : Logic  Operator=NOT  AllPortsSameDT=off  OutDataTypeStr=boolean
  Merge : Merge
  Switched : Subsystem  TreatAsAtomicUnit=on
  Out1 : Outport  VectorParamsAs1DForOutWhenUnconnected=off
  wires:
  In1/1 -> Average/1(In1), Switched/1(In1)
  Switched/1(Out1) -> Merge/1
  Average/1(Out1) -> Merge/2
  Merge/1 -> Out1/1
  Constant/1 -> Logical Operator/1, Switched/Enable
  Logical Operator/1 -> Average/Enable

== system TriphaseHardwaremodule/SMA_1delay_ratetrans ==
  u : Inport
  Delay : Delay  DelayLength=n_samples  InitialCondition=0  UseCircularBuffer=on
  Gain : Gain  Gain=1/n_samples
  Rate Transition : RateTransition  Integrity=off  InitialCondition=-1  OutPortSampleTime=SlowSampleTime
  Sum1 : Sum  Inputs=++-
  Unit Delay : UnitDelay  SampleTime=-1  HasFrameUpgradeWarning=on
  y : Outport  VectorParamsAs1DForOutWhenUnconnected=off
  wires:
  Gain/1 -> y/1
  Sum1/1 -> Unit Delay/1
  Delay/1 -> Sum1/3
  u/1 -> Sum1/2, Delay/1
  Unit Delay/1 -> Sum1/1, Rate Transition/1
  Rate Transition/1 -> Gain/1

== system TriphaseHardwaremodule/SMA_init0 ==
  u : Inport
  Delay : Delay  DelayLength=n_samples  InitialCondition=0  UseCircularBuffer=on
  Gain : Gain  Gain=1/n_samples
  Sum1 : Sum  Inputs=++-
  Unit Delay : UnitDelay  SampleTime=-1  HasFrameUpgradeWarning=on
  y : Outport  VectorParamsAs1DForOutWhenUnconnected=off
  wires:
  Unit Delay/1 -> Sum1/1
  u/1 -> Delay/1, Sum1/2
  Delay/1 -> Sum1/3
  Sum1/1 -> Unit Delay/1, Gain/1
  Gain/1 -> y/1

== system TriphaseHardwaremodule/adc ==
  x : Inport
  Constant1 : Constant  Value=ADC_Emulation  SampleTime=ControlSampleTime
  Discretize4 : Gain  Gain=(2^(MeasBits-1))  OutDataTypeStr=double  RndMeth=Round
  Multiport Switch : MultiPortSwitch  Inputs=2
  Normalize4 : Gain  Gain=1/MeasMax  OutDataTypeStr=double  RndMeth=Round
  Reexpand4 : Gain  Gain=MeasMax/(2^(MeasBits-1))  OutDataTypeStr=double  RndMeth=Round
  SMA_1delay_ratetrans : $bdroot/SMA_1delay_ratetrans  n_samples=round(ControlSampleTime/HWSampleTime)  SlowSampleTime=ControlSampleTime
  Saturate4 : Saturate  UpperLimit=1  LowerLimit=-1
  round4 : Rounding  Operator=round
  y : Outport  VectorParamsAs1DForOutWhenUnconnected=off
  wires:
  x/1 -> SMA_1delay_ratetrans/1
  Multiport Switch/1 -> y/1
  round4/1 -> Reexpand4/1
  Normalize4/1 -> Saturate4/1
  Saturate4/1 -> Discretize4/1
  Discretize4/1 -> round4/1
  SMA_1delay_ratetrans/1 -> Multiport Switch/2, Normalize4/1
  Reexpand4/1 -> Multiport Switch/3
  Constant1/1 -> Multiport Switch/1

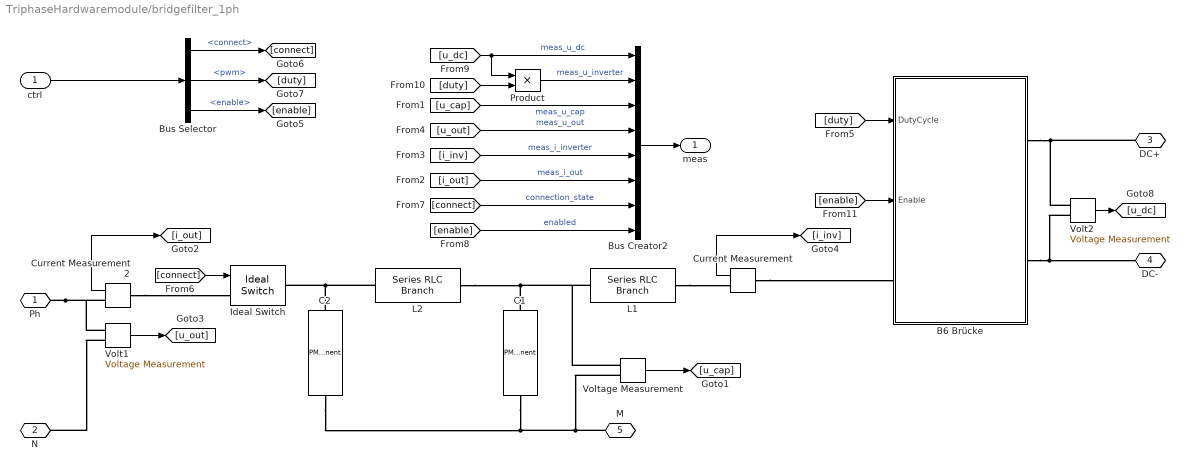
== system TriphaseHardwaremodule/bridgefilter_1ph ==
  ctrl : Inport
  B6 Brücke : Subsystem  LoadFcn=|  Variant=on
      | V_SIM_AVERAGE=Simulink.Variant('SIM_BRIDGE==SimBridgeMode.AVERAGE');
      | V_SIM_SWITCHED=Simulink.Variant('SIM_BRIDGE==SimBridgeMode.SWITCHED');
      settings: AttributesFormatString=%<ActiveVariant>
      settings: CopyFcn=|
      | V_SIM_AVERAGE=Simulink.Variant('SIM_BRIDGE==SimBridgeMode.AVERAGE');
      | V_SIM_SWITCHED=Simulink.Variant('SIM_BRIDGE==SimBridgeMode.SWITCHED');
  Bus Creator2 : BusCreator  Inputs=8
  Bus Selector : BusSelector  OutputSignals=connect,pwm,enable
  C1 : PMComponent  DialogController=POWERSYS.PowerSysDialog  LoadFcn=sps_rtmsupport('LoadFcn',gcbh);  StartFcn=sps_rtmsupport('StartFcn',gcbh);  StopFcn=sps_rtmsupport('StopFcn',gcbh);  PhysicalDomain=powersysdomain  LeftPortType=p1  RightPortType=p1  LConnTagsString=__new0  RConnTagsString=__new0  mask(Series RLC Branch){BranchType=RC, Resistance=R_C1, Inductance=L1, SetiL0=off, InitialCurrent=0, Capacitance=C1, Setx0=off, InitialVoltage=0, Measurements=None}
      mask prompts: BranchType "Branch type:"; Resistance "Resistance (Ohms):"; Inductance "Inductance (H):"; SetiL0 "Set the initial inductor current"; InitialCurrent "Inductor initial current (A):"; Capacitance "Capacitance (F):"; Setx0 "Set the initial capacitor voltage"; InitialVoltage "Capacitor initial voltage (V):"
      mask help:
      | Implements a series branch of RLC elements.
      | Use the 'Branch type' parameter to add or remove elements from the branch.
      mask init:
      | [s1,s2,s3,s4,r1,r2,l1,l2,c1,c2,c3,c4] = powericon('Series RLC Branch',Resistance,Inductance,Capacitance,BranchType);
      | powericon('RLCCback',gcb)
      | power_initmask();
      settings: CopyFcn=sps_rtmsupport('CopyFcn',gcbh);  DeleteFcn=sps_rtmsupport('DeleteFcn',gcbh);  UndoDeleteFcn=sps_rtmsupport('UndoDeleteFcn',gcbh);  ModelCloseFcn=sps_rtmsupport('ModelCloseFcn',gcbh);  PreSaveFcn=sps_rtmsupport('PreSaveFcn',gcbh);  PostSaveFcn=sps_rtmsupport('PostSaveFcn',gcbh);  NameChangeFcn=sps_rtmsupport('NameChangeFcn',gcbh);  PreCopyFcn=sps_rtmsupport('PreCopyFcn',gcbh);  OpenFcn=sps_rtmsupport('OpenFcn',gcbh, [1 4 7 9]);  CloseFcn=sps_rtmsupport('CloseFcn',gcbh);  PreDeleteFcn=sps_rtmsupport('PreDeleteFcn',gcbh);
      mask Help: helpview(psbhelp);
      mask TypeOptions BranchType: RLC | R | L | C | RL | RC | LC | Open circuit
      mask Callback BranchType: powericon('RLCCback',gcb)
      mask Callback Resistance: powericon('RLCCback',gcb)
      mask Callback Inductance: powericon('RLCCback',gcb)
      mask Callback SetiL0: powericon('RLCCback',gcb)
      mask Callback Capacitance: powericon('RLCCback',gcb)
      mask Callback Setx0: powericon('RLCCback',gcb)
      mask TypeOptions Measurements: None | Branch voltage | Branch current | Branch voltage and current
      mask Display:
      | plot(s1,s2,s3,s4,r1,r2,l1,l2,c1,c2,c3,c4)
      | color('red')
      | port_label('LConn',1,'+')
  C2 : PMComponent  DialogController=POWERSYS.PowerSysDialog  LoadFcn=sps_rtmsupport('LoadFcn',gcbh);  StartFcn=sps_rtmsupport('StartFcn',gcbh);  StopFcn=sps_rtmsupport('StopFcn',gcbh);  PhysicalDomain=powersysdomain  LeftPortType=p1  RightPortType=p1  LConnTagsString=__new0  RConnTagsString=__new0  mask(Series RLC Branch){BranchType=Open circuit, Resistance=R_C2, Inductance=L1, SetiL0=off, InitialCurrent=0, Capacitance=C2, Setx0=off, InitialVoltage=0, Measurements=None}
      mask prompts: BranchType "Branch type:"; Resistance "Resistance (Ohms):"; Inductance "Inductance (H):"; SetiL0 "Set the initial inductor current"; InitialCurrent "Inductor initial current (A):"; Capacitance "Capacitance (F):"; Setx0 "Set the initial capacitor voltage"; InitialVoltage "Capacitor initial voltage (V):"
      mask help:
      | Implements a series branch of RLC elements.
      | Use the 'Branch type' parameter to add or remove elements from the branch.
      mask init:
      | [s1,s2,s3,s4,r1,r2,l1,l2,c1,c2,c3,c4] = powericon('Series RLC Branch',Resistance,Inductance,Capacitance,BranchType);
      | powericon('RLCCback',gcb)
      | power_initmask();
      settings: CopyFcn=sps_rtmsupport('CopyFcn',gcbh);  DeleteFcn=sps_rtmsupport('DeleteFcn',gcbh);  UndoDeleteFcn=sps_rtmsupport('UndoDeleteFcn',gcbh);  ModelCloseFcn=sps_rtmsupport('ModelCloseFcn',gcbh);  PreSaveFcn=sps_rtmsupport('PreSaveFcn',gcbh);  PostSaveFcn=sps_rtmsupport('PostSaveFcn',gcbh);  NameChangeFcn=sps_rtmsupport('NameChangeFcn',gcbh);  PreCopyFcn=sps_rtmsupport('PreCopyFcn',gcbh);  OpenFcn=sps_rtmsupport('OpenFcn',gcbh, [1 4 7 9]);  CloseFcn=sps_rtmsupport('CloseFcn',gcbh);  PreDeleteFcn=sps_rtmsupport('PreDeleteFcn',gcbh);
      mask Help: helpview(psbhelp);
      mask TypeOptions BranchType: RLC | R | L | C | RL | RC | LC | Open circuit
      mask Callback BranchType: powericon('RLCCback',gcb)
      mask Callback Resistance: powericon('RLCCback',gcb)
      mask Callback Inductance: powericon('RLCCback',gcb)
      mask Callback SetiL0: powericon('RLCCback',gcb)
      mask Callback Capacitance: powericon('RLCCback',gcb)
      mask Callback Setx0: powericon('RLCCback',gcb)
      mask TypeOptions Measurements: None | Branch voltage | Branch current | Branch voltage and current
      mask Display:
      | plot(s1,s2,s3,s4,r1,r2,l1,l2,c1,c2,c3,c4)
      | color('red')
      | port_label('LConn',1,'+')
  Current Measurement : powerlib/Measurements/Current Measurement  PhasorSimulation=off  OutputType=Complex  PSBequivalent=0
      settings: SourceProductName=Simscape Electrical
  Current Measurement2 : powerlib/Measurements/Current Measurement  PhasorSimulation=off  OutputType=Complex  PSBequivalent=0
      settings: SourceProductName=Simscape Electrical
  Ideal Switch : powerlib/Power Electronics/Ideal Switch  Ron=0.001  Lon=0  IC=0  Rs=1e6  Cs=inf  Measurements=off
      settings: SourceProductName=Simscape Electrical
  L1 : powerlib/Elements/Series RLC Branch  LConnTagsString=__new0  RConnTagsString=__new0  BranchType=RL  Resistance=R_L1  Inductance=L1  SetiL0=off  InitialCurrent=0  Capacitance=1e-6  Setx0=off  InitialVoltage=0  Measurements=None
      settings: SourceProductName=Simscape Electrical
  L2 : powerlib/Elements/Series RLC Branch  LConnTagsString=__new0  RConnTagsString=__new0  BranchType=R  Resistance=0.001  Inductance=L2  SetiL0=off  InitialCurrent=0  Capacitance=1e-6  Setx0=off  InitialVoltage=0  Measurements=None
      settings: SourceProductName=Simscape Electrical
  Product : Product
  Volt1 : powerlib/Measurements/Voltage Measurement  PhasorSimulation=off  OutputType=Complex  PSBequivalent=0
      settings: SourceProductName=Simscape Electrical
  Volt2 : powerlib/Measurements/Voltage Measurement  PhasorSimulation=off  OutputType=Complex  PSBequivalent=0
      settings: SourceProductName=Simscape Electrical
  Voltage Measurement : powerlib/Measurements/Voltage Measurement  PhasorSimulation=off  OutputType=Complex  PSBequivalent=0
      settings: SourceProductName=Simscape Electrical
  Ph : PMIOPort  Side=Left
  N : PMIOPort  Port=2  Side=Left
  DC+ : PMIOPort  Port=3  Side=Right
  DC- : PMIOPort  Port=4  Side=Right
  M : PMIOPort  Port=5  Side=Right
  meas : Outport  VectorParamsAs1DForOutWhenUnconnected=off
  wires:
  Volt2/1 -> [u_dc]
  Bus Selector/2 -> [duty]  "<pwm>"
  Bus Selector/1 -> [connect]  "<connect>"
  [connect] -> Bus Creator2/7  "connection_state"
  ctrl/1 -> Bus Selector/1
  [i_out] -> Bus Creator2/6  "meas_i_out"
  [i_inv] -> Bus Creator2/5  "meas_i_inverter"
  [u_out] -> Bus Creator2/4  "meas_u_out"
  [u_cap] -> Bus Creator2/3  "meas_u_cap"
  Current Measurement2/1 -> [i_out]
  Volt1/1 -> [u_out]
  [connect] -> Ideal Switch/1
  Bus Selector/3 -> [enable]  "<enable>"
  [enable] -> Bus Creator2/8  "enabled"
  Bus Creator2/1 -> meas/1
  [u_dc] -> Bus Creator2/1, Product/1  "meas_u_dc"
  [duty] -> B6 Brücke/1(DutyCycle)
  [enable] -> B6 Brücke/2(Enable)
  Current Measurement/1 -> [i_inv]
  Voltage Measurement/1 -> [u_cap]
  Product/1 -> Bus Creator2/2  "meas_u_inverter"
  [duty] -> Product/2
  connections:
  Current Measurement/LConn1 -- B6 Brücke/LConn1
  L2/LConn1 -- C2/LConn1 -- Ideal Switch/RConn1
  Volt2/LConn2 -- B6 Brücke/RConn2 -- DC-/RConn1
  DC+/RConn1 -- B6 Brücke/RConn1 -- Volt2/LConn1
  Ph/RConn1 -- Volt1/LConn1 -- Current Measurement2/RConn1
  Current Measurement2/LConn1 -- Ideal Switch/LConn1
  Volt1/LConn2 -- N/RConn1
  Voltage Measurement/LConn2 -- C2/RConn1 -- C1/RConn1 -- M/RConn1
  L2/RConn1 -- C1/LConn1 -- Voltage Measurement/LConn1 -- L1/LConn1
  L1/RConn1 -- Current Measurement/RConn1

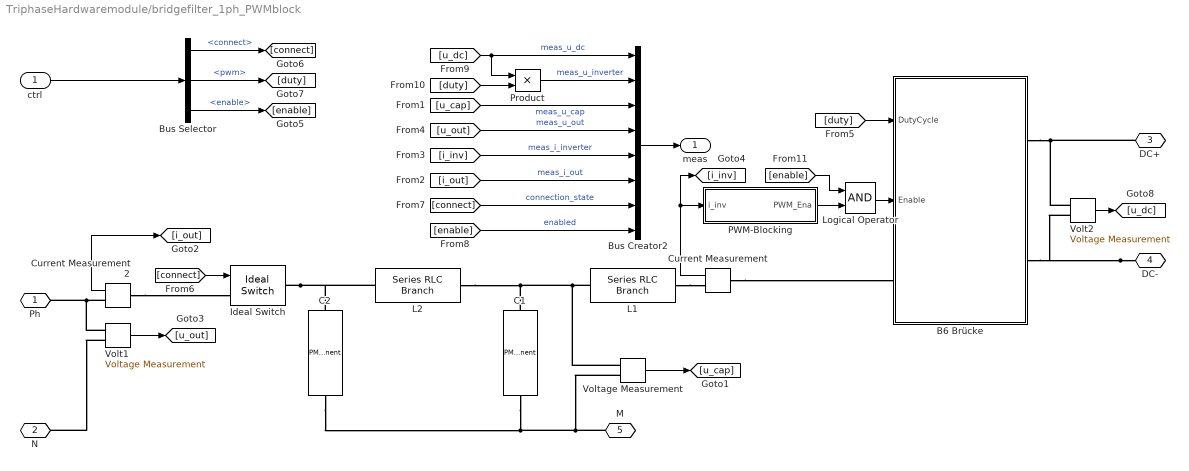
== system TriphaseHardwaremodule/bridgefilter_1ph_PWMblock ==
  ctrl : Inport
  B6 Brücke : Subsystem  LoadFcn=|  Variant=on
      | V_SIM_AVERAGE=Simulink.Variant('SIM_BRIDGE==SimBridgeMode.AVERAGE');
      | V_SIM_SWITCHED=Simulink.Variant('SIM_BRIDGE==SimBridgeMode.SWITCHED');
      settings: AttributesFormatString=%<ActiveVariant>
      settings: CopyFcn=|
      | V_SIM_AVERAGE=Simulink.Variant('SIM_BRIDGE==SimBridgeMode.AVERAGE');
      | V_SIM_SWITCHED=Simulink.Variant('SIM_BRIDGE==SimBridgeMode.SWITCHED');
  Bus Creator2 : BusCreator  Inputs=8
  Bus Selector : BusSelector  OutputSignals=connect,pwm,enable
  C1 : PMComponent  DialogController=POWERSYS.PowerSysDialog  LoadFcn=sps_rtmsupport('LoadFcn',gcbh);  StartFcn=sps_rtmsupport('StartFcn',gcbh);  StopFcn=sps_rtmsupport('StopFcn',gcbh);  PhysicalDomain=powersysdomain  LeftPortType=p1  RightPortType=p1  LConnTagsString=__new0  RConnTagsString=__new0  mask(Series RLC Branch){BranchType=RC, Resistance=R_C1, Inductance=L1, SetiL0=off, InitialCurrent=0, Capacitance=C1, Setx0=off, InitialVoltage=0, Measurements=None}
      mask prompts: BranchType "Branch type:"; Resistance "Resistance (Ohms):"; Inductance "Inductance (H):"; SetiL0 "Set the initial inductor current"; InitialCurrent "Inductor initial current (A):"; Capacitance "Capacitance (F):"; Setx0 "Set the initial capacitor voltage"; InitialVoltage "Capacitor initial voltage (V):"
      mask help:
      | Implements a series branch of RLC elements.
      | Use the 'Branch type' parameter to add or remove elements from the branch.
      mask init:
      | [s1,s2,s3,s4,r1,r2,l1,l2,c1,c2,c3,c4] = powericon('Series RLC Branch',Resistance,Inductance,Capacitance,BranchType);
      | powericon('RLCCback',gcb)
      | power_initmask();
      settings: CopyFcn=sps_rtmsupport('CopyFcn',gcbh);  DeleteFcn=sps_rtmsupport('DeleteFcn',gcbh);  UndoDeleteFcn=sps_rtmsupport('UndoDeleteFcn',gcbh);  ModelCloseFcn=sps_rtmsupport('ModelCloseFcn',gcbh);  PreSaveFcn=sps_rtmsupport('PreSaveFcn',gcbh);  PostSaveFcn=sps_rtmsupport('PostSaveFcn',gcbh);  NameChangeFcn=sps_rtmsupport('NameChangeFcn',gcbh);  PreCopyFcn=sps_rtmsupport('PreCopyFcn',gcbh);  OpenFcn=sps_rtmsupport('OpenFcn',gcbh, [1 4 7 9]);  CloseFcn=sps_rtmsupport('CloseFcn',gcbh);  PreDeleteFcn=sps_rtmsupport('PreDeleteFcn',gcbh);
      mask Help: helpview(psbhelp);
      mask TypeOptions BranchType: RLC | R | L | C | RL | RC | LC | Open circuit
      mask Callback BranchType: powericon('RLCCback',gcb)
      mask Callback Resistance: powericon('RLCCback',gcb)
      mask Callback Inductance: powericon('RLCCback',gcb)
      mask Callback SetiL0: powericon('RLCCback',gcb)
      mask Callback Capacitance: powericon('RLCCback',gcb)
      mask Callback Setx0: powericon('RLCCback',gcb)
      mask TypeOptions Measurements: None | Branch voltage | Branch current | Branch voltage and current
      mask Display:
      | plot(s1,s2,s3,s4,r1,r2,l1,l2,c1,c2,c3,c4)
      | color('red')
      | port_label('LConn',1,'+')
  C2 : PMComponent  DialogController=POWERSYS.PowerSysDialog  LoadFcn=sps_rtmsupport('LoadFcn',gcbh);  StartFcn=sps_rtmsupport('StartFcn',gcbh);  StopFcn=sps_rtmsupport('StopFcn',gcbh);  PhysicalDomain=powersysdomain  LeftPortType=p1  RightPortType=p1  LConnTagsString=__new0  RConnTagsString=__new0  mask(Series RLC Branch){BranchType=Open circuit, Resistance=R_C2, Inductance=L1, SetiL0=off, InitialCurrent=0, Capacitance=C2, Setx0=off, InitialVoltage=0, Measurements=None}
      mask prompts: BranchType "Branch type:"; Resistance "Resistance (Ohms):"; Inductance "Inductance (H):"; SetiL0 "Set the initial inductor current"; InitialCurrent "Inductor initial current (A):"; Capacitance "Capacitance (F):"; Setx0 "Set the initial capacitor voltage"; InitialVoltage "Capacitor initial voltage (V):"
      mask help:
      | Implements a series branch of RLC elements.
      | Use the 'Branch type' parameter to add or remove elements from the branch.
      mask init:
      | [s1,s2,s3,s4,r1,r2,l1,l2,c1,c2,c3,c4] = powericon('Series RLC Branch',Resistance,Inductance,Capacitance,BranchType);
      | powericon('RLCCback',gcb)
      | power_initmask();
      settings: CopyFcn=sps_rtmsupport('CopyFcn',gcbh);  DeleteFcn=sps_rtmsupport('DeleteFcn',gcbh);  UndoDeleteFcn=sps_rtmsupport('UndoDeleteFcn',gcbh);  ModelCloseFcn=sps_rtmsupport('ModelCloseFcn',gcbh);  PreSaveFcn=sps_rtmsupport('PreSaveFcn',gcbh);  PostSaveFcn=sps_rtmsupport('PostSaveFcn',gcbh);  NameChangeFcn=sps_rtmsupport('NameChangeFcn',gcbh);  PreCopyFcn=sps_rtmsupport('PreCopyFcn',gcbh);  OpenFcn=sps_rtmsupport('OpenFcn',gcbh, [1 4 7 9]);  CloseFcn=sps_rtmsupport('CloseFcn',gcbh);  PreDeleteFcn=sps_rtmsupport('PreDeleteFcn',gcbh);
      mask Help: helpview(psbhelp);
      mask TypeOptions BranchType: RLC | R | L | C | RL | RC | LC | Open circuit
      mask Callback BranchType: powericon('RLCCback',gcb)
      mask Callback Resistance: powericon('RLCCback',gcb)
      mask Callback Inductance: powericon('RLCCback',gcb)
      mask Callback SetiL0: powericon('RLCCback',gcb)
      mask Callback Capacitance: powericon('RLCCback',gcb)
      mask Callback Setx0: powericon('RLCCback',gcb)
      mask TypeOptions Measurements: None | Branch voltage | Branch current | Branch voltage and current
      mask Display:
      | plot(s1,s2,s3,s4,r1,r2,l1,l2,c1,c2,c3,c4)
      | color('red')
      | port_label('LConn',1,'+')
  Current Measurement : powerlib/Measurements/Current Measurement  PhasorSimulation=off  OutputType=Complex  PSBequivalent=0
      settings: SourceProductName=Simscape Electrical
  Current Measurement2 : powerlib/Measurements/Current Measurement  PhasorSimulation=off  OutputType=Complex  PSBequivalent=0
      settings: SourceProductName=Simscape Electrical
  Ideal Switch : powerlib/Power Electronics/Ideal Switch  Ron=0.001  Lon=0  IC=0  Rs=1e6  Cs=inf  Measurements=off
      settings: SourceProductName=Simscape Electrical
  L1 : powerlib/Elements/Series RLC Branch  LConnTagsString=__new0  RConnTagsString=__new0  BranchType=RL  Resistance=R_L1  Inductance=L1  SetiL0=off  InitialCurrent=0  Capacitance=1e-6  Setx0=off  InitialVoltage=0  Measurements=None
      settings: SourceProductName=Simscape Electrical
  L2 : powerlib/Elements/Series RLC Branch  LConnTagsString=__new0  RConnTagsString=__new0  BranchType=R  Resistance=0.001  Inductance=L2  SetiL0=off  InitialCurrent=0  Capacitance=1e-6  Setx0=off  InitialVoltage=0  Measurements=None
      settings: SourceProductName=Simscape Electrical
  Logical Operator : Logic  AllPortsSameDT=off  OutDataTypeStr=boolean
  PWM-Blocking : Subsystem
  Product : Product
  Volt1 : powerlib/Measurements/Voltage Measurement  PhasorSimulation=off  OutputType=Complex  PSBequivalent=0
      settings: SourceProductName=Simscape Electrical
  Volt2 : powerlib/Measurements/Voltage Measurement  PhasorSimulation=off  OutputType=Complex  PSBequivalent=0
      settings: SourceProductName=Simscape Electrical
  Voltage Measurement : powerlib/Measurements/Voltage Measurement  PhasorSimulation=off  OutputType=Complex  PSBequivalent=0
      settings: SourceProductName=Simscape Electrical
  Ph : PMIOPort  Side=Left
  N : PMIOPort  Port=2  Side=Left
  DC+ : PMIOPort  Port=3  Side=Right
  DC- : PMIOPort  Port=4  Side=Right
  M : PMIOPort  Port=5  Side=Right
  meas : Outport  VectorParamsAs1DForOutWhenUnconnected=off
  wires:
  [duty] -> Product/2
  Product/1 -> Bus Creator2/2  "meas_u_inverter"
  Voltage Measurement/1 -> [u_cap]
  Current Measurement/1 -> PWM-Blocking/1("i_inv\t"), [i_inv]
  Logical Operator/1 -> B6 Brücke/2(Enable)
  [duty] -> B6 Brücke/1(DutyCycle)
  [u_dc] -> Product/1, Bus Creator2/1  "meas_u_dc"
  Bus Creator2/1 -> meas/1
  [enable] -> Bus Creator2/8  "enabled"
  Bus Selector/3 -> [enable]  "<enable>"
  [connect] -> Ideal Switch/1
  Volt1/1 -> [u_out]
  Current Measurement2/1 -> [i_out]
  [u_cap] -> Bus Creator2/3  "meas_u_cap"
  [u_out] -> Bus Creator2/4  "meas_u_out"
  [i_inv] -> Bus Creator2/5  "meas_i_inverter"
  [i_out] -> Bus Creator2/6  "meas_i_out"
  ctrl/1 -> Bus Selector/1
  [connect] -> Bus Creator2/7  "connection_state"
  Bus Selector/1 -> [connect]  "<connect>"
  Bus Selector/2 -> [duty]  "<pwm>"
  Volt2/1 -> [u_dc]
  [enable] -> Logical Operator/1
  PWM-Blocking/1(PWM_Ena) -> Logical Operator/2
  connections:
  L1/RConn1 -- Current Measurement/RConn1
  L1/LConn1 -- Voltage Measurement/LConn1 -- C1/LConn1 -- L2/RConn1
  M/RConn1 -- C1/RConn1 -- C2/RConn1 -- Voltage Measurement/LConn2
  Volt1/LConn2 -- N/RConn1
  Current Measurement2/LConn1 -- Ideal Switch/LConn1
  Current Measurement2/RConn1 -- Volt1/LConn1 -- Ph/RConn1
  Volt2/LConn1 -- B6 Brücke/RConn1 -- DC+/RConn1
  DC-/RConn1 -- B6 Brücke/RConn2 -- Volt2/LConn2
  Ideal Switch/RConn1 -- C2/LConn1 -- L2/LConn1
  Current Measurement/LConn1 -- B6 Brücke/LConn1

== system TriphaseHardwaremodule/ctrlSelect2 ==
  ctrl : Inport
  Bus Creator1 : BusCreator  Inputs=3
  Bus Creator3 : BusCreator  Inputs=3
  Bus Selector : BusSelector  OutputSignals=pwm,connect,enable
  Data Type Conversion : DataTypeConversion  OutDataTypeStr=boolean
  Rate Transition : RateTransition  Integrity=off  Deterministic=off  OutPortSampleTime=0
  Selector1 : Selector  InputPortWidth=2  IndexOptions=Index vector (dialog)  Indices=[1]  OutputSizes=1
  Selector2 : Selector  InputPortWidth=2  IndexOptions=Index vector (dialog)  Indices=2  OutputSizes=1
  Sum of Elements : Sum  Inputs=+
  Sum of Elements1 : Sum  Inputs=+  SampleTime=ControlSampleTime
  ctrl1 : Outport  VectorParamsAs1DForOutWhenUnconnected=off
  ctrl2 : Outport  Port=2  VectorParamsAs1DForOutWhenUnconnected=off
  wires:
  Rate Transition/1 -> Selector1/1, Selector2/1
  Bus Selector/2 -> Sum of Elements/1  "<connect>"
  Data Type Conversion/1 -> Bus Creator1/3, Bus Creator3/3  "enable"
  Selector1/1 -> Bus Creator1/1  "pwm"
  Bus Creator3/1 -> ctrl2/1
  Selector2/1 -> Bus Creator3/1  "pwm"
  Sum of Elements/1 -> Bus Creator1/2, Bus Creator3/2  "connect"
  Bus Creator1/1 -> ctrl1/1
  ctrl/1 -> Bus Selector/1
  Bus Selector/3 -> Sum of Elements1/1  "<enable>"
  Bus Selector/1 -> Rate Transition/1  "<pwm>"
  Sum of Elements1/1 -> Data Type Conversion/1  "enable"

== system TriphaseHardwaremodule/ctrlSelect3 ==
  ctrl : Inport
  Bus Creator1 : BusCreator  Inputs=3
  Bus Creator2 : BusCreator  Inputs=3
  Bus Creator3 : BusCreator  Inputs=3
  Bus Selector : BusSelector  OutputSignals=pwm,connect,enable
  Data Type Conversion : DataTypeConversion  OutDataTypeStr=boolean
  Rate Transition : RateTransition  Integrity=off  Deterministic=off  OutPortSampleTime=0
  Selector1 : Selector  InputPortWidth=3  IndexOptions=Index vector (dialog)  Indices=[1]  OutputSizes=1
  Selector2 : Selector  InputPortWidth=3  IndexOptions=Index vector (dialog)  Indices=2  OutputSizes=1
  Selector3 : Selector  InputPortWidth=3  IndexOptions=Index vector (dialog)  Indices=3  OutputSizes=1
  Sum of Elements : Sum  Inputs=+
  Sum of Elements1 : Sum  Inputs=+  SampleTime=ControlSampleTime
  ctrl1 : Outport  VectorParamsAs1DForOutWhenUnconnected=off
  ctrl2 : Outport  Port=2  VectorParamsAs1DForOutWhenUnconnected=off
  ctrl3 : Outport  Port=3  VectorParamsAs1DForOutWhenUnconnected=off
  wires:
  Bus Selector/1 -> Rate Transition/1  "<pwm>"
  Selector3/1 -> Bus Creator2/1  "pwm"
  Bus Creator2/1 -> ctrl3/1
  Bus Selector/3 -> Sum of Elements1/1  "<enable>"
  ctrl/1 -> Bus Selector/1
  Bus Creator1/1 -> ctrl1/1
  Sum of Elements/1 -> Bus Creator1/2, Bus Creator2/2, Bus Creator3/2  "connect"
  Selector2/1 -> Bus Creator3/1  "pwm"
  Bus Creator3/1 -> ctrl2/1
  Selector1/1 -> Bus Creator1/1  "pwm"
  Sum of Elements1/1 -> Data Type Conversion/1  "enable"
  Bus Selector/2 -> Sum of Elements/1  "<connect>"
  Rate Transition/1 -> Selector2/1, Selector3/1, Selector1/1
  Data Type Conversion/1 -> Bus Creator1/3, Bus Creator2/3, Bus Creator3/3  "enable"
